simulink model "cell_station_2017_327_constant_load_for_battery_limit_suc"  (R2016b)
settings: Solver=VariableStepAuto  StartTime=0.0  StopTime=120*2  FixedStep=1e-6  RelTol=1e-3
undefined symbols (not defined in the file or in its folder): Acid, Lead, magnitude
libraries: powerlib x33, simulink x16, electricdrivelib x1
(part 1 of 2)
settings Model: Creator=Ray Hu  LastModifiedBy=Administrator

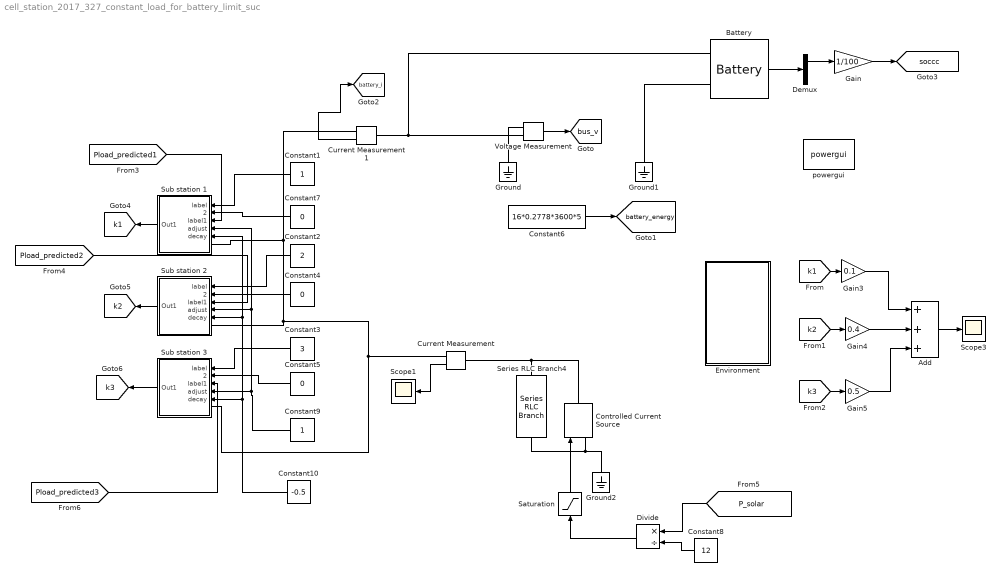
== system cell_station_2017_327_constant_load_for_battery_limit_suc ==
  Add : Sum  Inputs=+++
  Battery : electricdrivelib/Extra Sources/Battery  BatType=Lead-Acid  ShowTempParam=off  ThermalPreset=no  NomV=12  NomQ=0.2778*5  SOC=80  Batt_Tr=1  PresetModel=off  MaxQ=1.4469  MinV=9  FullV=13.0658  Dis_rate=10  R=0.086393  Normal_OP=0.2778*5  expZone="[12.2171      0.00463]"  current=[6.5 13 32.5]  Units=Time  Tci=20  NomT=25  T2=0  MaxQ2=2.208  FullV2=3.45  Normal_OP2=2.8  expZone2="[3.22        0.23]"  Rca=0.6  ti=1000  Dp=0
  Constant1 : Constant
  Constant10 : Constant  Value=-0.5
  Constant2 : Constant  Value=2
  Constant3 : Constant  Value=3
  Constant4 : Constant  Value=0
  Constant5 : Constant  Value=0
  Constant6 : Constant  Value=16*0.2778*3600*5
  Constant7 : Constant  Value=0
  Constant8 : Constant  Value=12
  Constant9 : Constant
  Controlled Current Source : powerlib/Electrical Sources/Controlled Current Source  Initialize=on  Source_Type=AC  Amplitude=0  Phase=0  Frequency=0  Measurements=None
  Current Measurement : powerlib/Measurements/Current Measurement  PhasorSimulation=off  OutputType=Complex  PSBequivalent=0
  Current Measurement1 : powerlib/Measurements/Current Measurement  PhasorSimulation=off  OutputType=Complex  PSBequivalent=0
  Demux : Demux  Outputs=3
  Divide : Product  Inputs=*/
  Environment : Subsystem
  Gain : Gain  Gain=1/100
  Gain3 : Gain  Gain=0.1
  Gain4 : Gain  Gain=0.4
  Gain5 : Gain  Gain=0.5
  Ground : powerlib/Elements/Ground  LConnTagsString=a
  Ground1 : powerlib/Elements/Ground  LConnTagsString=a
  Ground2 : powerlib/Elements/Ground  LConnTagsString=a
  Saturation : Saturate  UpperLimit=inf  LowerLimit=0
  Scope1 : Scope
  Scope3 : Scope
  Series RLC Branch4 : powerlib/Elements/Series RLC Branch  LConnTagsString=__new0  RConnTagsString=__new0  BranchType=C  Resistance=10  Inductance=1e-3  SetiL0=off  InitialCurrent=0  Capacitance=1e-6  Setx0=on  InitialVoltage=12  Measurements=None
  Sub station 1 : Subsystem
  Sub station 2 : Subsystem
  Sub station 3 : Subsystem
  Voltage Measurement : powerlib/Measurements/Voltage Measurement  PhasorSimulation=off  OutputType=Complex  PSBequivalent=0
  powergui : powerlib/powergui  Priority=1  SimulationMode=Continuous  SolverType=Tustin/Backward Euler (TBE)  SampleTime=50e-5  frequency=60  SPID=off  DisableSnubberDevices=off  DisableRonSwitches=off  DisableVfSwitches=off  SwTol=0  DisplayEquations=off  Interpol=off  ExternalGateDelay=off  methode=off  Ts=10  FunctionMessages=off  echomessages=off  HookPort=off  EnableUseOfTLC=off  x0status=blocks  frequencyindice=0  Pbase=100e6  ErrMax=1e-4  Iterations=50  UnitsV=kV  UnitsW=MW  buscounter=0  RestoreLinks=warning  ResistiveCurrentMeasurement=off  Frange=[0:2:500]  Ylog=off  Xlog=on  ShowGrid=off  save=off  variable=ZData  structure=0  ZoomFFT=off  StartTime=0.0  cycles=1  DisplayStyle=1  fundamental=60  FreqAxis=off  MaxFrequency=1000  frequencyindicesteady=1  RmsSteady=1  display=off
  tag scope: battery_energy=global, battery_i=global, bus_v=global, k1=global, k2=global, k3=global, soccc=global
  wires:
  Current Measurement/1 -> Scope1/1
  Voltage Measurement/1 -> [bus_v]
  Current Measurement1/1 -> [battery_i]
  Constant1/1 -> Sub station 1/1(label)
  Constant2/1 -> Sub station 2/1(label)
  Constant3/1 -> Sub station 3/1(label)
  Demux/1 -> Gain/1
  Constant4/1 -> Sub station 2/2(test_sig)
  Constant5/1 -> Sub station 3/2(test_sig)
  Constant6/1 -> [battery_energy]
  [k3] -> Gain5/1
  [k2] -> Gain4/1
  [k1] -> Gain3/1
  Gain4/1 -> Add/2
  Gain3/1 -> Add/1
  Gain5/1 -> Add/3
  Add/1 -> Scope3/1
  Constant7/1 -> Sub station 1/2(test_sig)
  Battery/1 -> Demux/1
  Sub station 1/1(Out1) -> [k1]
  Sub station 2/1(Out1) -> [k2]
  Sub station 3/1(Out1) -> [k3]
  [P_solar] -> Divide/1
  Constant8/1 -> Divide/2
  Divide/1 -> Saturation/1
  Saturation/1 -> Controlled Current Source/1
  [Pload_predicted1] -> Sub station 1/3(label1)
  [Pload_predicted2] -> Sub station 2/3(label1)
  [Pload_predicted3] -> Sub station 3/3(label1)
  Constant9/1 -> Sub station 3/4(adjust), Sub station 2/4(adjust), Sub station 1/4(adjust)
  Constant10/1 -> Sub station 3/5(decay), Sub station 2/5(decay), Sub station 1/5(decay)
  Gain/1 -> [soccc]
  connections:
  Voltage Measurement/LConn2 -- Ground/LConn1
  Current Measurement/RConn1 -- Sub station 3/LConn1 -- Sub station 2/LConn1 -- Sub station 1/LConn1 -- Current Measurement1/RConn1
  Controlled Current Source/RConn1 -- Series RLC Branch4/LConn1 -- Current Measurement/LConn1
  Ground1/LConn1 -- Battery/LConn2
  Current Measurement1/LConn1 -- Battery/LConn1 -- Voltage Measurement/LConn1
  Ground2/LConn1 -- Series RLC Branch4/RConn1 -- Controlled Current Source/LConn1

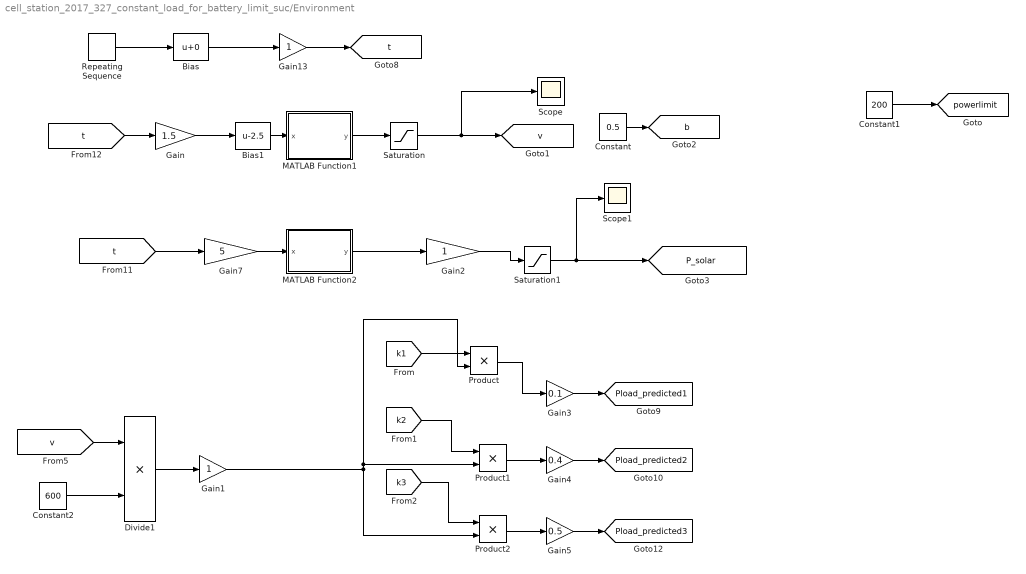
== system cell_station_2017_327_constant_load_for_battery_limit_suc/Environment ==
  Bias : Bias
  Bias1 : Bias  Bias=-2.5
  Constant : Constant  Value=0.5
  Constant1 : Constant  Value=200
  Constant2 : Constant  Value=600
  Divide1 : Product  Inputs=**
  Gain : Gain  Gain=1.5
  Gain1 : Gain
  Gain13 : Gain
  Gain2 : Gain
  Gain3 : Gain  Gain=0.1
  Gain4 : Gain  Gain=0.4
  Gain5 : Gain  Gain=0.5
  Gain7 : Gain  Gain=5
  MATLAB Function1 : MATLAB Function  TreatAsAtomicUnit=on
  MATLAB Function2 : MATLAB Function  TreatAsAtomicUnit=on
  Product : Product
  Product1 : Product
  Product2 : Product
  Repeating Sequence : simulink/Sources/Repeating Sequence  rep_seq_t=[0 120]  rep_seq_y=[0 24]
  Saturation : Saturate  UpperLimit=1  LowerLimit=0
  Saturation1 : Saturate  UpperLimit=inf  LowerLimit=0
  Scope : Scope
  Scope1 : Scope
  tag scope: P_solar=global, Pload_predicted1=global, Pload_predicted2=global, Pload_predicted3=global, b=global, powerlimit=global, t=global, v=global
  wires:
  Gain7/1 -> MATLAB Function2/1(x)
  MATLAB Function2/1(y) -> Gain2/1
  Bias/1 -> Gain13/1
  Saturation1/1 -> [P_solar], Scope1/1
  Gain13/1 -> [t]
  Repeating Sequence/1 -> Bias/1
  [t] -> Gain7/1
  MATLAB Function1/1(y) -> Saturation/1
  Gain/1 -> Bias1/1
  [t] -> Gain/1
  [v] -> Divide1/1
  Constant2/1 -> Divide1/2
  Divide1/1 -> Gain1/1
  Gain1/1 -> Product2/2, Product/2, Product1/2
  Gain3/1 -> [Pload_predicted1]
  Gain4/1 -> [Pload_predicted2]
  Gain5/1 -> [Pload_predicted3]
  Saturation/1 -> Scope/1, [v]
  Constant/1 -> [b]
  [k1] -> Product/1
  Product/1 -> Gain3/1
  [k3] -> Product2/1
  Product2/1 -> Gain5/1
  Product1/1 -> Gain4/1
  [k2] -> Product1/1
  Gain2/1 -> Saturation1/1
  Constant1/1 -> [powerlimit]
  Bias1/1 -> MATLAB Function1/1(x)

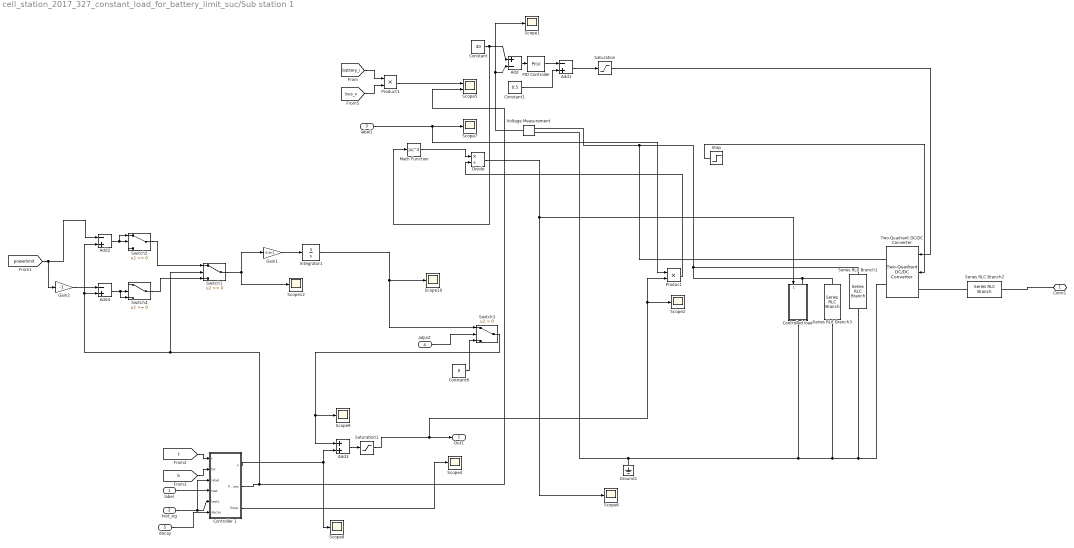
== system cell_station_2017_327_constant_load_for_battery_limit_suc/Sub station 1 ==
  label : Inport
  test_sig : Inport  Port=2
  label1 : Inport  Port=3
  adjust : Inport  Port=4
  decay : Inport  Port=5
  Add : Sum  Inputs=+-
  Add1 : Sum  Inputs=-+
  Add2 : Sum  Inputs=-+
  Add3 : Sum
  Add4 : Sum  Inputs=-+
  Constant : Constant  Value=40
  Constant1 : Constant  Value=0.5
  Constant6 : Constant  Value=0
  Controlled load : Subsystem
  Controller 1 : Subsystem
  Divide : Product  Inputs=*/
  Gain1 : Gain  Gain=-0.5e-2
  Gain2 : Gain  Gain=-1
  Ground1 : powerlib/Elements/Ground  LConnTagsString=a
  Integrator1 : Integrator
  Math Function : Math  Operator=magnitude^2  SaturateOnIntegerOverflow=on
  PID Controller : simulink/Continuous/PID Controller  Controller=PI  TimeDomain=Continuous-time  SampleTime=-1  IntegratorMethod=Forward Euler  FilterMethod=Forward Euler  Form=Parallel  UseFilter=on  ControllerParametersSource=internal  P=1e-5  I=0.1  D=0  N=100  InitialConditionSource=internal  InitialConditionForIntegrator=0  InitialConditionForFilter=0  ExternalReset=none  LimitOutput=off  UpperSaturationLimit=inf  LowerSaturationLimit=-inf  LinearizeAsGain=on  AntiWindupMode=none  Kb=1  TrackingMode=off  Kt=1  PParamMin=[]  PParamMax=[]  IParamMin=[]  IParamMax=[]  DParamMin=[]  DParamMax=[]  NParamMin=[]  NParamMax=[]  KbParamMin=[]  KbParamMax=[]  KtParamMin=[]  KtParamMax=[]  POutMin=[]  POutMax=[]  IOutMin=[]  IOutMax=[]  DOutMin=[]  DOutMax=[]  NOutMin=[]  NOutMax=[]  KbOutMin=[]  KbOutMax=[]  KtOutMin=[]  KtOutMax=[]  IntegratorOutMin=[]  IntegratorOutMax=[]  FilterOutMin=[]  FilterOutMax=[]  SumOutMin=[]  SumOutMax=[]  SumI1OutMin=[]  SumI1OutMax=[]  SumI2OutMin=[]  SumI2OutMax=[]  SumI3OutMin=[]  SumI3OutMax=[]  SumDOutMin=[]  SumDOutMax=[]  SaturationOutMin=[]  SaturationOutMax=[]  IntegratorContinuousStateAttributes=''  IntegratorStateMustResolveToSignalObject=off  IntegratorRTWStateStorageClass=Auto  FilterContinuousStateAttributes=''  FilterStateMustResolveToSignalObject=off  FilterRTWStateStorageClass=Auto  DifferentiatorICPrevScaledInput=0  DifferentiatorOutMin=[]  DifferentiatorOutMax=[]
  Product : Product
  Product1 : Product
  Saturation : Saturate  UpperLimit=0.9  LowerLimit=0.1
  Saturation1 : Saturate  UpperLimit=1  LowerLimit=0.1
  Scope{1..2,4,6..10,12} (9 alike) : Scope
  Scope5 : Scope  NumInputPorts=2
  Series RLC Branch1 : powerlib/Elements/Series RLC Branch  LConnTagsString=__new0  RConnTagsString=__new0  BranchType=C  Resistance=10  Inductance=1e-3  SetiL0=off  InitialCurrent=0  Capacitance=1e-6  Setx0=on  InitialVoltage=20  Measurements=None
  Series RLC Branch2 : powerlib/Elements/Series RLC Branch  LConnTagsString=__new0  RConnTagsString=__new0  BranchType=L  Resistance=10  Inductance=1e-3  SetiL0=off  InitialCurrent=0  Capacitance=1e-6  Setx0=off  InitialVoltage=0  Measurements=None
  Series RLC Branch3 : powerlib/Elements/Series RLC Branch  LConnTagsString=__new0  RConnTagsString=__new0  BranchType=R  Resistance=100  Inductance=1e-3  SetiL0=off  InitialCurrent=0  Capacitance=1e-6  Setx0=on  InitialVoltage=60  Measurements=None
  Step : Step  Time=0  Before=1  After=0  SampleTime=0
  Switch1 : Switch
  Switch2 : Switch
  Switch3 : Switch  Criteria=u2 > Threshold
  Switch4 : Switch
  Two-Quadrant DC/DC Converter : powerlib/Power Electronics/Two-Quadrant DC//DC Converter  ModelType=Average model (D-controlled)  Ron=1e-3  Rs=1e6  Cs=inf  Vforward=[0,0]  Ron_Diode=1e-3  Rs_Diode=1e6  Cs_Diode=inf  Vf_Diode=1e-3  Rs_CurrentSource=inf
  Voltage Measurement : powerlib/Measurements/Voltage Measurement  PhasorSimulation=off  OutputType=Complex  PSBequivalent=0
  Conn1 : PMIOPort  Port=1  Side=Left
  Out1 : Outport
  wires:
  Add1/1 -> Saturation/1
  Constant1/1 -> Add1/2
  PID Controller/1 -> Add1/1
  Step/1 -> Two-Quadrant DC/DC Converter/2
  Saturation/1 -> Two-Quadrant DC/DC Converter/1
  Add/1 -> PID Controller/1
  Voltage Measurement/1 -> Scope1/1, Add/2
  label1/1 -> Product/1, Scope7/1
  Product/1 -> Divide/2
  [t] -> Controller 1/1(t)
  [b] -> Controller 1/2(b0)
  label/1 -> Controller 1/3(label)
  Controller 1/3(Estar) -> Scope4/1
  Divide/1 -> Controlled load/1(Controllerd_R), Scope6/1
  Math Function/1 -> Divide/1
  Constant/1 -> Math Function/1, Add/1
  [battery_i] -> Product1/1
  [bus_v] -> Product1/2
  Product1/1 -> Scope5/1
  test_sig/1 -> Controller 1/5(test1), Controller 1/4(test)
  Controller 1/1("k ") -> Scope8/1, Add3/2
  Add3/1 -> Saturation1/1
  Saturation1/1 -> Product/2, Scope2/1, Out1/1
  decay/1 -> Controller 1/6(decay)
  Switch3/1 -> Scope9/1, Add3/1
  Gain1/1 -> Integrator1/1
  adjust/1 -> Switch3/2
  Integrator1/1 -> Switch3/1, Scope10/1
  [powerlimit] -> Gain2/1, Add2/1
  Switch1/1 -> Gain1/1, Scope12/1
  Constant6/1 -> Switch3/3
  Switch2/1 -> Switch1/1
  Switch4/1 -> Switch1/3
  Gain2/1 -> Add4/1
  Controller 1/2(P_guess) -> Switch1/2, Add2/2, Add4/2, Scope5/2
  Add2/1 -> Switch2/1, Switch2/2
  Add4/1 -> Switch4/3, Switch4/2
  connections:
  Conn1/RConn1 -- Series RLC Branch2/LConn1
  Series RLC Branch1/RConn1 -- Voltage Measurement/LConn2 -- Ground1/LConn1 -- Controlled load/RConn1 -- Series RLC Branch3/RConn1 -- Two-Quadrant DC/DC Converter/RConn2
  Series RLC Branch2/RConn1 -- Two-Quadrant DC/DC Converter/LConn1
  Series RLC Branch1/LConn1 -- Controlled load/LConn1 -- Series RLC Branch3/LConn1 -- Voltage Measurement/LConn1 -- Two-Quadrant DC/DC Converter/RConn1

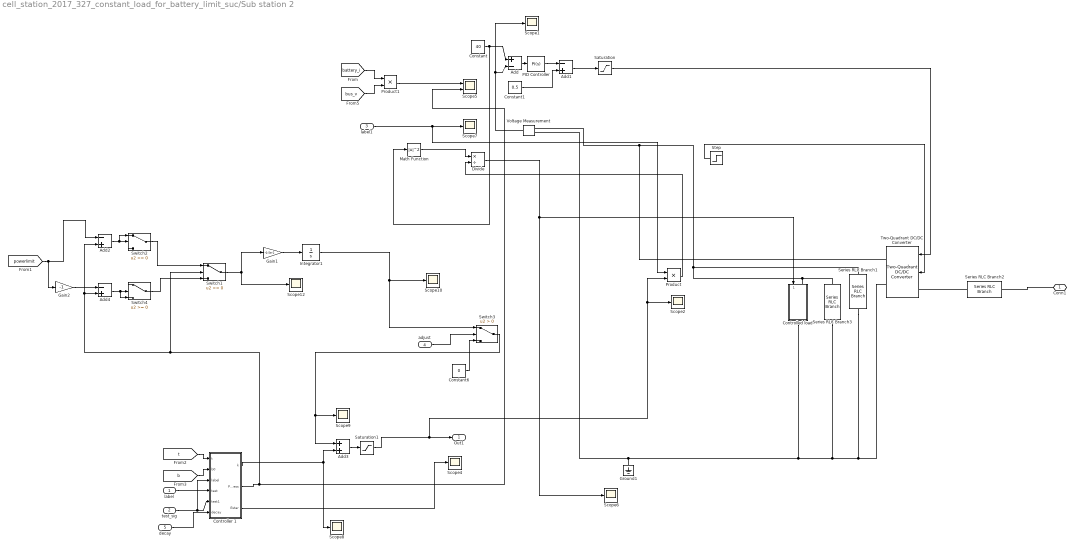
== system cell_station_2017_327_constant_load_for_battery_limit_suc/Sub station 2 ==
  label : Inport
  test_sig : Inport  Port=2
  label1 : Inport  Port=3
  adjust : Inport  Port=4
  decay : Inport  Port=5
  Add : Sum  Inputs=+-
  Add1 : Sum  Inputs=-+
  Add2 : Sum  Inputs=-+
  Add3 : Sum
  Add4 : Sum  Inputs=-+
  Constant : Constant  Value=40
  Constant1 : Constant  Value=0.5
  Constant6 : Constant  Value=0
  Controlled load : Subsystem
  Controller 1 : Subsystem
  Divide : Product  Inputs=*/
  Gain1 : Gain  Gain=-0.5e-2
  Gain2 : Gain  Gain=-1
  Ground1 : powerlib/Elements/Ground  LConnTagsString=a
  Integrator1 : Integrator
  Math Function : Math  Operator=magnitude^2  SaturateOnIntegerOverflow=on
  PID Controller : simulink/Continuous/PID Controller  Controller=PI  TimeDomain=Continuous-time  SampleTime=-1  IntegratorMethod=Forward Euler  FilterMethod=Forward Euler  Form=Parallel  UseFilter=on  ControllerParametersSource=internal  P=1e-5  I=0.1  D=0  N=100  InitialConditionSource=internal  InitialConditionForIntegrator=0  InitialConditionForFilter=0  ExternalReset=none  LimitOutput=off  UpperSaturationLimit=inf  LowerSaturationLimit=-inf  LinearizeAsGain=on  AntiWindupMode=none  Kb=1  TrackingMode=off  Kt=1  PParamMin=[]  PParamMax=[]  IParamMin=[]  IParamMax=[]  DParamMin=[]  DParamMax=[]  NParamMin=[]  NParamMax=[]  KbParamMin=[]  KbParamMax=[]  KtParamMin=[]  KtParamMax=[]  POutMin=[]  POutMax=[]  IOutMin=[]  IOutMax=[]  DOutMin=[]  DOutMax=[]  NOutMin=[]  NOutMax=[]  KbOutMin=[]  KbOutMax=[]  KtOutMin=[]  KtOutMax=[]  IntegratorOutMin=[]  IntegratorOutMax=[]  FilterOutMin=[]  FilterOutMax=[]  SumOutMin=[]  SumOutMax=[]  SumI1OutMin=[]  SumI1OutMax=[]  SumI2OutMin=[]  SumI2OutMax=[]  SumI3OutMin=[]  SumI3OutMax=[]  SumDOutMin=[]  SumDOutMax=[]  SaturationOutMin=[]  SaturationOutMax=[]  IntegratorContinuousStateAttributes=''  IntegratorStateMustResolveToSignalObject=off  IntegratorRTWStateStorageClass=Auto  FilterContinuousStateAttributes=''  FilterStateMustResolveToSignalObject=off  FilterRTWStateStorageClass=Auto  DifferentiatorICPrevScaledInput=0  DifferentiatorOutMin=[]  DifferentiatorOutMax=[]
  Product : Product
  Product1 : Product
  Saturation : Saturate  UpperLimit=0.9  LowerLimit=0.1
  Saturation1 : Saturate  UpperLimit=1  LowerLimit=0.1
  Scope{1..2,4,6..10,12} (9 alike) : Scope
  Scope5 : Scope  NumInputPorts=2
  Series RLC Branch1 : powerlib/Elements/Series RLC Branch  LConnTagsString=__new0  RConnTagsString=__new0  BranchType=C  Resistance=10  Inductance=1e-3  SetiL0=off  InitialCurrent=0  Capacitance=1e-6  Setx0=on  InitialVoltage=20  Measurements=None
  Series RLC Branch2 : powerlib/Elements/Series RLC Branch  LConnTagsString=__new0  RConnTagsString=__new0  BranchType=L  Resistance=10  Inductance=1e-3  SetiL0=off  InitialCurrent=0  Capacitance=1e-6  Setx0=off  InitialVoltage=0  Measurements=None
  Series RLC Branch3 : powerlib/Elements/Series RLC Branch  LConnTagsString=__new0  RConnTagsString=__new0  BranchType=R  Resistance=100  Inductance=1e-3  SetiL0=off  InitialCurrent=0  Capacitance=1e-6  Setx0=on  InitialVoltage=60  Measurements=None
  Step : Step  Time=0  Before=1  After=0  SampleTime=0
  Switch1 : Switch
  Switch2 : Switch
  Switch3 : Switch  Criteria=u2 > Threshold
  Switch4 : Switch
  Two-Quadrant DC/DC Converter : powerlib/Power Electronics/Two-Quadrant DC//DC Converter  ModelType=Average model (D-controlled)  Ron=1e-3  Rs=1e6  Cs=inf  Vforward=[0,0]  Ron_Diode=1e-3  Rs_Diode=1e6  Cs_Diode=inf  Vf_Diode=1e-3  Rs_CurrentSource=inf
  Voltage Measurement : powerlib/Measurements/Voltage Measurement  PhasorSimulation=off  OutputType=Complex  PSBequivalent=0
  Conn1 : PMIOPort  Port=1  Side=Left
  Out1 : Outport
  wires:
  Add1/1 -> Saturation/1
  Constant1/1 -> Add1/2
  PID Controller/1 -> Add1/1
  Step/1 -> Two-Quadrant DC/DC Converter/2
  Saturation/1 -> Two-Quadrant DC/DC Converter/1
  Add/1 -> PID Controller/1
  Voltage Measurement/1 -> Scope1/1, Add/2
  label1/1 -> Product/1, Scope7/1
  Product/1 -> Divide/2
  [t] -> Controller 1/1(t)
  [b] -> Controller 1/2(b0)
  label/1 -> Controller 1/3(label)
  Controller 1/3(Estar) -> Scope4/1
  Divide/1 -> Controlled load/1(Controllerd_R), Scope6/1
  Math Function/1 -> Divide/1
  Constant/1 -> Math Function/1, Add/1
  [battery_i] -> Product1/1
  [bus_v] -> Product1/2
  Product1/1 -> Scope5/1
  test_sig/1 -> Controller 1/5(test1), Controller 1/4(test)
  Controller 1/1("k ") -> Scope8/1, Add3/2
  Add3/1 -> Saturation1/1
  Saturation1/1 -> Product/2, Scope2/1, Out1/1
  decay/1 -> Controller 1/6(decay)
  Switch3/1 -> Scope9/1, Add3/1
  Gain1/1 -> Integrator1/1
  adjust/1 -> Switch3/2
  Integrator1/1 -> Switch3/1, Scope10/1
  [powerlimit] -> Gain2/1, Add2/1
  Switch1/1 -> Gain1/1, Scope12/1
  Constant6/1 -> Switch3/3
  Switch2/1 -> Switch1/1
  Switch4/1 -> Switch1/3
  Gain2/1 -> Add4/1
  Controller 1/2(P_guess) -> Switch1/2, Add2/2, Add4/2, Scope5/2
  Add2/1 -> Switch2/1, Switch2/2
  Add4/1 -> Switch4/3, Switch4/2
  connections:
  Conn1/RConn1 -- Series RLC Branch2/LConn1
  Series RLC Branch1/RConn1 -- Voltage Measurement/LConn2 -- Ground1/LConn1 -- Controlled load/RConn1 -- Series RLC Branch3/RConn1 -- Two-Quadrant DC/DC Converter/RConn2
  Series RLC Branch2/RConn1 -- Two-Quadrant DC/DC Converter/LConn1
  Series RLC Branch1/LConn1 -- Controlled load/LConn1 -- Series RLC Branch3/LConn1 -- Voltage Measurement/LConn1 -- Two-Quadrant DC/DC Converter/RConn1

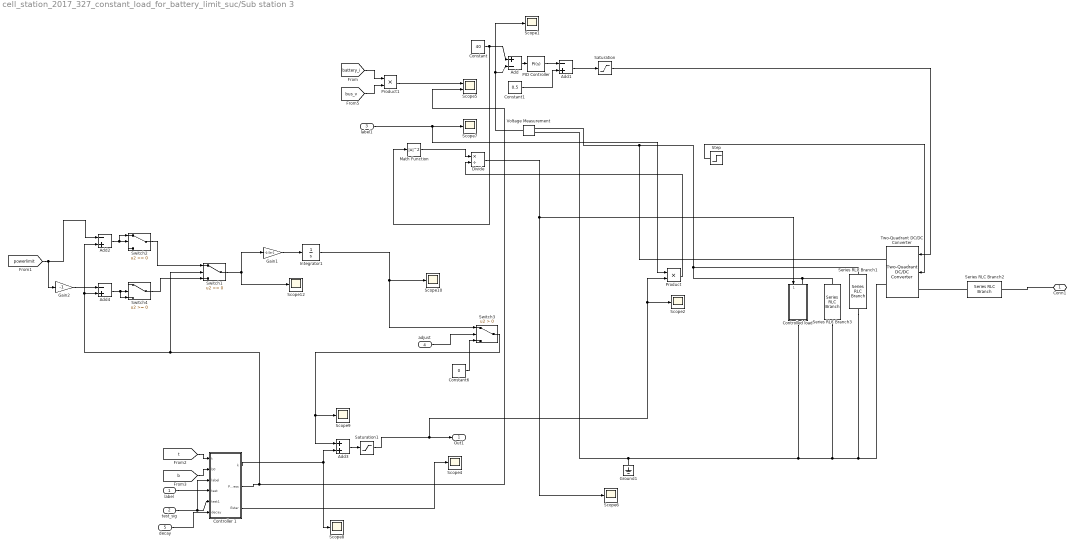
== system cell_station_2017_327_constant_load_for_battery_limit_suc/Sub station 3 ==
  label : Inport
  test_sig : Inport  Port=2
  label1 : Inport  Port=3
  adjust : Inport  Port=4
  decay : Inport  Port=5
  Add : Sum  Inputs=+-
  Add1 : Sum  Inputs=-+
  Add2 : Sum  Inputs=-+
  Add3 : Sum
  Add4 : Sum  Inputs=-+
  Constant : Constant  Value=40
  Constant1 : Constant  Value=0.5
  Constant6 : Constant  Value=0
  Controlled load : Subsystem
  Controller 1 : Subsystem
  Divide : Product  Inputs=*/
  Gain1 : Gain  Gain=-0.5e-2
  Gain2 : Gain  Gain=-1
  Ground1 : powerlib/Elements/Ground  LConnTagsString=a
  Integrator1 : Integrator
  Math Function : Math  Operator=magnitude^2  SaturateOnIntegerOverflow=on
  PID Controller : simulink/Continuous/PID Controller  Controller=PI  TimeDomain=Continuous-time  SampleTime=-1  IntegratorMethod=Forward Euler  FilterMethod=Forward Euler  Form=Parallel  UseFilter=on  ControllerParametersSource=internal  P=1e-5  I=0.1  D=0  N=100  InitialConditionSource=internal  InitialConditionForIntegrator=0  InitialConditionForFilter=0  ExternalReset=none  LimitOutput=off  UpperSaturationLimit=inf  LowerSaturationLimit=-inf  LinearizeAsGain=on  AntiWindupMode=none  Kb=1  TrackingMode=off  Kt=1  PParamMin=[]  PParamMax=[]  IParamMin=[]  IParamMax=[]  DParamMin=[]  DParamMax=[]  NParamMin=[]  NParamMax=[]  KbParamMin=[]  KbParamMax=[]  KtParamMin=[]  KtParamMax=[]  POutMin=[]  POutMax=[]  IOutMin=[]  IOutMax=[]  DOutMin=[]  DOutMax=[]  NOutMin=[]  NOutMax=[]  KbOutMin=[]  KbOutMax=[]  KtOutMin=[]  KtOutMax=[]  IntegratorOutMin=[]  IntegratorOutMax=[]  FilterOutMin=[]  FilterOutMax=[]  SumOutMin=[]  SumOutMax=[]  SumI1OutMin=[]  SumI1OutMax=[]  SumI2OutMin=[]  SumI2OutMax=[]  SumI3OutMin=[]  SumI3OutMax=[]  SumDOutMin=[]  SumDOutMax=[]  SaturationOutMin=[]  SaturationOutMax=[]  IntegratorContinuousStateAttributes=''  IntegratorStateMustResolveToSignalObject=off  IntegratorRTWStateStorageClass=Auto  FilterContinuousStateAttributes=''  FilterStateMustResolveToSignalObject=off  FilterRTWStateStorageClass=Auto  DifferentiatorICPrevScaledInput=0  DifferentiatorOutMin=[]  DifferentiatorOutMax=[]
  Product : Product
  Product1 : Product
  Saturation : Saturate  UpperLimit=0.9  LowerLimit=0.1
  Saturation1 : Saturate  UpperLimit=1  LowerLimit=0.1
  Scope{1..2,4,6..10,12} (9 alike) : Scope
  Scope5 : Scope  NumInputPorts=2
  Series RLC Branch1 : powerlib/Elements/Series RLC Branch  LConnTagsString=__new0  RConnTagsString=__new0  BranchType=C  Resistance=10  Inductance=1e-3  SetiL0=off  InitialCurrent=0  Capacitance=1e-6  Setx0=on  InitialVoltage=20  Measurements=None
  Series RLC Branch2 : powerlib/Elements/Series RLC Branch  LConnTagsString=__new0  RConnTagsString=__new0  BranchType=L  Resistance=10  Inductance=1e-3  SetiL0=off  InitialCurrent=0  Capacitance=1e-6  Setx0=off  InitialVoltage=0  Measurements=None
  Series RLC Branch3 : powerlib/Elements/Series RLC Branch  LConnTagsString=__new0  RConnTagsString=__new0  BranchType=R  Resistance=100  Inductance=1e-3  SetiL0=off  InitialCurrent=0  Capacitance=1e-6  Setx0=on  InitialVoltage=60  Measurements=None
  Step : Step  Time=0  Before=1  After=0  SampleTime=0
  Switch1 : Switch
  Switch2 : Switch
  Switch3 : Switch  Criteria=u2 > Threshold
  Switch4 : Switch
  Two-Quadrant DC/DC Converter : powerlib/Power Electronics/Two-Quadrant DC//DC Converter  ModelType=Average model (D-controlled)  Ron=1e-3  Rs=1e6  Cs=inf  Vforward=[0,0]  Ron_Diode=1e-3  Rs_Diode=1e6  Cs_Diode=inf  Vf_Diode=1e-3  Rs_CurrentSource=inf
  Voltage Measurement : powerlib/Measurements/Voltage Measurement  PhasorSimulation=off  OutputType=Complex  PSBequivalent=0
  Conn1 : PMIOPort  Port=1  Side=Left
  Out1 : Outport
  wires:
  Add1/1 -> Saturation/1
  Constant1/1 -> Add1/2
  PID Controller/1 -> Add1/1
  Step/1 -> Two-Quadrant DC/DC Converter/2
  Saturation/1 -> Two-Quadrant DC/DC Converter/1
  Add/1 -> PID Controller/1
  Voltage Measurement/1 -> Scope1/1, Add/2
  label1/1 -> Product/1, Scope7/1
  Product/1 -> Divide/2
  [t] -> Controller 1/1(t)
  [b] -> Controller 1/2(b0)
  label/1 -> Controller 1/3(label)
  Controller 1/3(Estar) -> Scope4/1
  Divide/1 -> Controlled load/1(Controllerd_R), Scope6/1
  Math Function/1 -> Divide/1
  Constant/1 -> Math Function/1, Add/1
  [battery_i] -> Product1/1
  [bus_v] -> Product1/2
  Product1/1 -> Scope5/1
  test_sig/1 -> Controller 1/5(test1), Controller 1/4(test)
  Controller 1/1("k ") -> Scope8/1, Add3/2
  Add3/1 -> Saturation1/1
  Saturation1/1 -> Product/2, Scope2/1, Out1/1
  decay/1 -> Controller 1/6(decay)
  Switch3/1 -> Scope9/1, Add3/1
  Gain1/1 -> Integrator1/1
  adjust/1 -> Switch3/2
  Integrator1/1 -> Switch3/1, Scope10/1
  [powerlimit] -> Gain2/1, Add2/1
  Switch1/1 -> Gain1/1, Scope12/1
  Constant6/1 -> Switch3/3
  Switch2/1 -> Switch1/1
  Switch4/1 -> Switch1/3
  Gain2/1 -> Add4/1
  Controller 1/2(P_guess) -> Switch1/2, Add2/2, Add4/2, Scope5/2
  Add2/1 -> Switch2/1, Switch2/2
  Add4/1 -> Switch4/3, Switch4/2
  connections:
  Conn1/RConn1 -- Series RLC Branch2/LConn1
  Series RLC Branch1/RConn1 -- Voltage Measurement/LConn2 -- Ground1/LConn1 -- Controlled load/RConn1 -- Series RLC Branch3/RConn1 -- Two-Quadrant DC/DC Converter/RConn2
  Series RLC Branch2/RConn1 -- Two-Quadrant DC/DC Converter/LConn1
  Series RLC Branch1/LConn1 -- Controlled load/LConn1 -- Series RLC Branch3/LConn1 -- Voltage Measurement/LConn1 -- Two-Quadrant DC/DC Converter/RConn1

== system cell_station_2017_327_constant_load_for_battery_limit_suc/Sub station 1/Controlled load ==
  Controllerd_R : Inport
  Controlled Current Source : powerlib/Electrical Sources/Controlled Current Source  Initialize=on  Source_Type=DC  Amplitude=0  Phase=0  Frequency=0  Measurements=None
  Divide : Product  Inputs=*/
  Saturation : Saturate  UpperLimit=inf  LowerLimit=0.1
  Voltage Measurement : powerlib/Measurements/Voltage Measurement  PhasorSimulation=off  OutputType=Complex  PSBequivalent=0
  Conn1 : PMIOPort  Port=1  Side=Left
  Conn2 : PMIOPort  Port=2  Side=Right
  wires:
  Voltage Measurement/1 -> Divide/1
  Controllerd_R/1 -> Saturation/1
  Divide/1 -> Controlled Current Source/1
  Saturation/1 -> Divide/2
  connections:
  Voltage Measurement/LConn2 -- Controlled Current Source/RConn1 -- Conn2/RConn1
  Voltage Measurement/LConn1 -- Controlled Current Source/LConn1 -- Conn1/RConn1

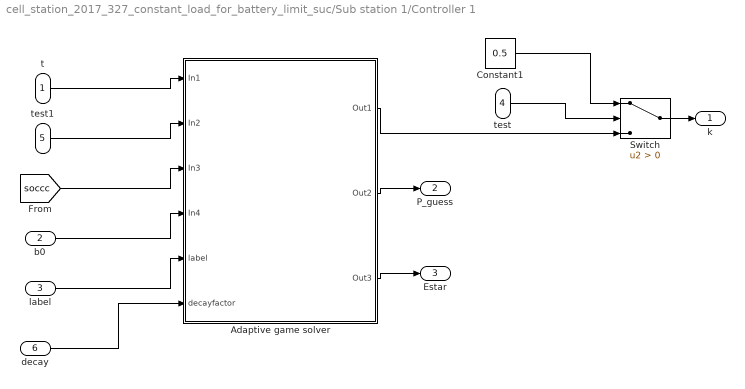
== system cell_station_2017_327_constant_load_for_battery_limit_suc/Sub station 1/Controller 1 ==
  t : Inport
  b0 : Inport  Port=2
  label : Inport  Port=3
  test : Inport  Port=4
  test1 : Inport  Port=5
  decay : Inport  Port=6
  Adaptive game solver : Subsystem
  Constant1 : Constant  Value=0.5
  Switch : Switch  Criteria=u2 > Threshold
  "k " : Outport
  P_guess : Outport  Port=2
  Estar : Outport  Port=3
  wires:
  Constant1/1 -> Switch/1
  Switch/1 -> "k "/1
  test/1 -> Switch/2
  t/1 -> Adaptive game solver/1(In1)
  test1/1 -> Adaptive game solver/2(In2)
  [soccc] -> Adaptive game solver/3(In3)
  b0/1 -> Adaptive game solver/4(In4)
  label/1 -> Adaptive game solver/5(label)
  Adaptive game solver/1(Out1) -> Switch/3
  Adaptive game solver/2(Out2) -> P_guess/1
  Adaptive game solver/3(Out3) -> Estar/1
  decay/1 -> Adaptive game solver/6(decayfactor)

== system cell_station_2017_327_constant_load_for_battery_limit_suc/Sub station 2/Controlled load ==
  Controllerd_R : Inport
  Controlled Current Source : powerlib/Electrical Sources/Controlled Current Source  Initialize=on  Source_Type=DC  Amplitude=0  Phase=0  Frequency=0  Measurements=None
  Divide : Product  Inputs=*/
  Saturation : Saturate  UpperLimit=inf  LowerLimit=0.1
  Voltage Measurement : powerlib/Measurements/Voltage Measurement  PhasorSimulation=off  OutputType=Complex  PSBequivalent=0
  Conn1 : PMIOPort  Port=1  Side=Left
  Conn2 : PMIOPort  Port=2  Side=Right
  wires:
  Voltage Measurement/1 -> Divide/1
  Controllerd_R/1 -> Saturation/1
  Divide/1 -> Controlled Current Source/1
  Saturation/1 -> Divide/2
  connections:
  Voltage Measurement/LConn2 -- Controlled Current Source/RConn1 -- Conn2/RConn1
  Voltage Measurement/LConn1 -- Controlled Current Source/LConn1 -- Conn1/RConn1

== system cell_station_2017_327_constant_load_for_battery_limit_suc/Sub station 2/Controller 1 ==
  t : Inport
  b0 : Inport  Port=2
  label : Inport  Port=3
  test : Inport  Port=4
  test1 : Inport  Port=5
  decay : Inport  Port=6
  Adaptive game solver : Subsystem
  Constant1 : Constant  Value=0.5
  Switch : Switch  Criteria=u2 > Threshold
  "k " : Outport
  P_guess : Outport  Port=2
  Estar : Outport  Port=3
  wires:
  Constant1/1 -> Switch/1
  Switch/1 -> "k "/1
  test/1 -> Switch/2
  t/1 -> Adaptive game solver/1(In1)
  test1/1 -> Adaptive game solver/2(In2)
  [soccc] -> Adaptive game solver/3(In3)
  b0/1 -> Adaptive game solver/4(In4)
  label/1 -> Adaptive game solver/5(label)
  Adaptive game solver/1(Out1) -> Switch/3
  Adaptive game solver/2(Out2) -> P_guess/1
  Adaptive game solver/3(Out3) -> Estar/1
  decay/1 -> Adaptive game solver/6(decayfactor)

== system cell_station_2017_327_constant_load_for_battery_limit_suc/Sub station 3/Controlled load ==
  Controllerd_R : Inport
  Controlled Current Source : powerlib/Electrical Sources/Controlled Current Source  Initialize=on  Source_Type=DC  Amplitude=0  Phase=0  Frequency=0  Measurements=None
  Divide : Product  Inputs=*/
  Saturation : Saturate  UpperLimit=inf  LowerLimit=0.1
  Voltage Measurement : powerlib/Measurements/Voltage Measurement  PhasorSimulation=off  OutputType=Complex  PSBequivalent=0
  Conn1 : PMIOPort  Port=1  Side=Left
  Conn2 : PMIOPort  Port=2  Side=Right
  wires:
  Voltage Measurement/1 -> Divide/1
  Controllerd_R/1 -> Saturation/1
  Divide/1 -> Controlled Current Source/1
  Saturation/1 -> Divide/2
  connections:
  Voltage Measurement/LConn2 -- Controlled Current Source/RConn1 -- Conn2/RConn1
  Voltage Measurement/LConn1 -- Controlled Current Source/LConn1 -- Conn1/RConn1

== system cell_station_2017_327_constant_load_for_battery_limit_suc/Sub station 3/Controller 1 ==
  t : Inport
  b0 : Inport  Port=2
  label : Inport  Port=3
  test : Inport  Port=4
  test1 : Inport  Port=5
  decay : Inport  Port=6
  Adaptive game solver : Subsystem
  Constant1 : Constant  Value=0.5
  Switch : Switch  Criteria=u2 > Threshold
  "k " : Outport
  P_guess : Outport  Port=2
  Estar : Outport  Port=3
  wires:
  Constant1/1 -> Switch/1
  Switch/1 -> "k "/1
  test/1 -> Switch/2
  t/1 -> Adaptive game solver/1(In1)
  test1/1 -> Adaptive game solver/2(In2)
  [soccc] -> Adaptive game solver/3(In3)
  b0/1 -> Adaptive game solver/4(In4)
  label/1 -> Adaptive game solver/5(label)
  Adaptive game solver/1(Out1) -> Switch/3
  Adaptive game solver/2(Out2) -> P_guess/1
  Adaptive game solver/3(Out3) -> Estar/1
  decay/1 -> Adaptive game solver/6(decayfactor)

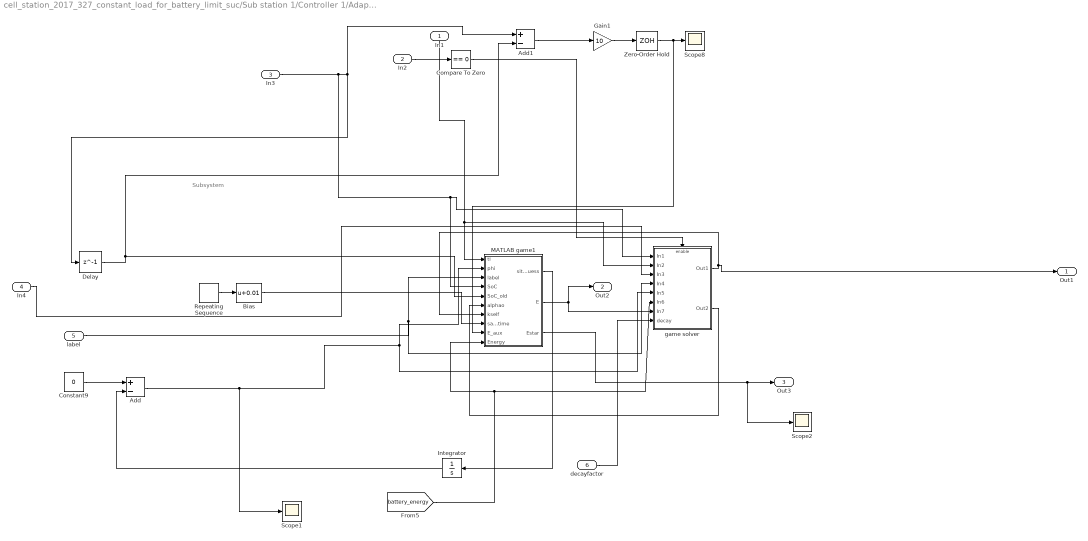
== system cell_station_2017_327_constant_load_for_battery_limit_suc/Sub station 1/Controller 1/Adaptive game solver ==
  note: Subsystem
  In1 : Inport
  In2 : Inport  Port=2
  In3 : Inport  Port=3
  In4 : Inport  Port=4
  label : Inport  Port=5
  decayfactor : Inport  Port=6
  Add : Sum  Inputs=+-
  Add1 : Sum  Inputs=+-
  Bias : Bias  Bias=0.01
  Compare To Zero : simulink/Logic and Bit Operations/Compare To Zero  relop===  OutDataTypeStr=boolean
  Constant9 : Constant  Value=0
  Delay : Delay  DelayLength=1  InitialCondition=0  SampleTime=0.1
  Gain1 : Gain  Gain=10
  Integrator : Integrator
  MATLAB game1 : MATLAB Function  TreatAsAtomicUnit=on
      settings: MinAlgLoopOccurrences=on
  Repeating Sequence : simulink/Sources/Repeating Sequence  rep_seq_t=[0 0.5]  rep_seq_y=[0 0.5]
  Scope1 : Scope
  Scope2 : Scope
  Scope8 : Scope
  Zero-Order Hold : ZeroOrderHold  SampleTime=0.1
  game solver : Subsystem
  Out1 : Outport
  Out2 : Outport  Port=2
  Out3 : Outport  Port=3
  wires:
  game solver/2(Out2) -> MATLAB game1/6(alphao)
  Constant9/1 -> Add/1
  Repeating Sequence/1 -> Bias/1
  Add1/1 -> Gain1/1
  Gain1/1 -> Zero-Order Hold/1
  In2/1 -> Compare To Zero/1
  Compare To Zero/1 -> game solver/Enable
  [battery_energy] -> MATLAB game1/10(Energy), game solver/6(In6)
  Bias/1 -> MATLAB game1/8(sampletime)
  label/1 -> game solver/4(In4), MATLAB game1/3(label)
  Add/1 -> Scope1/1, game solver/5(In5), MATLAB game1/2(phi)
  In1/1 -> MATLAB game1/1(ti), game solver/2(In2)
  In4/1 -> game solver/3(In3)
  Integrator/1 -> Add/2
  MATLAB game1/1(sitaguess) -> Integrator/1
  Delay/1 -> MATLAB game1/5(SoC_old), Add1/2
  Zero-Order Hold/1 -> MATLAB game1/9(E_aux), Scope8/1
  MATLAB game1/2(E) -> game solver/7(In7), Out2/1
  game solver/1(Out1) -> Out1/1, MATLAB game1/7(kself)
  In3/1 -> game solver/1(In1), MATLAB game1/4(SoC), Add1/1, Delay/1
  MATLAB game1/3(Estar) -> Scope2/1, Out3/1
  decayfactor/1 -> game solver/8(decay)

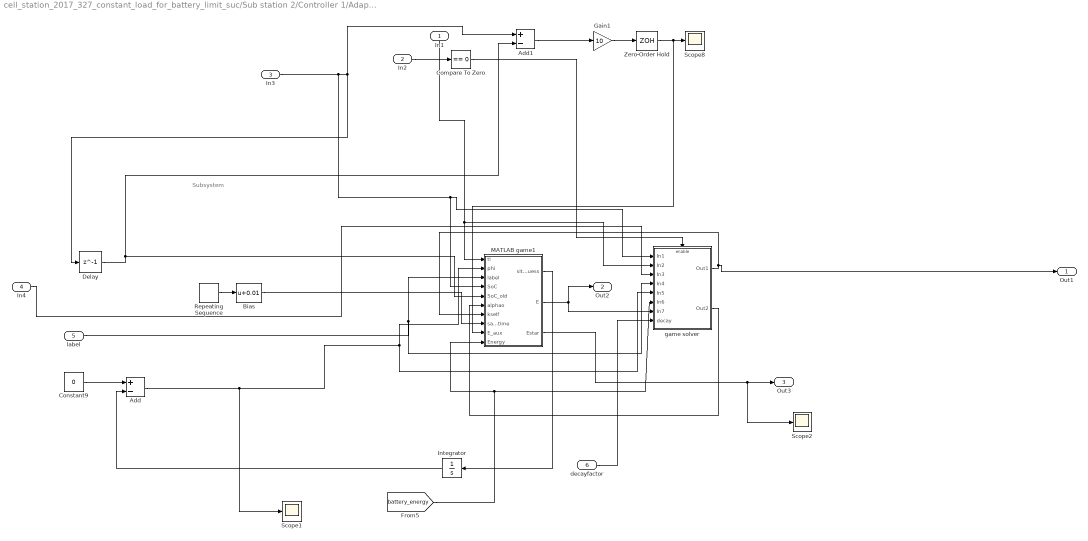
== system cell_station_2017_327_constant_load_for_battery_limit_suc/Sub station 2/Controller 1/Adaptive game solver ==
  note: Subsystem
  In1 : Inport
  In2 : Inport  Port=2
  In3 : Inport  Port=3
  In4 : Inport  Port=4
  label : Inport  Port=5
  decayfactor : Inport  Port=6
  Add : Sum  Inputs=+-
  Add1 : Sum  Inputs=+-
  Bias : Bias  Bias=0.01
  Compare To Zero : simulink/Logic and Bit Operations/Compare To Zero  relop===  OutDataTypeStr=boolean
  Constant9 : Constant  Value=0
  Delay : Delay  DelayLength=1  InitialCondition=0  SampleTime=0.1
  Gain1 : Gain  Gain=10
  Integrator : Integrator
  MATLAB game1 : MATLAB Function  TreatAsAtomicUnit=on
      settings: MinAlgLoopOccurrences=on
  Repeating Sequence : simulink/Sources/Repeating Sequence  rep_seq_t=[0 0.5]  rep_seq_y=[0 0.5]
  Scope1 : Scope
  Scope2 : Scope
  Scope8 : Scope
  Zero-Order Hold : ZeroOrderHold  SampleTime=0.1
  game solver : Subsystem
  Out1 : Outport
  Out2 : Outport  Port=2
  Out3 : Outport  Port=3
  wires:
  game solver/2(Out2) -> MATLAB game1/6(alphao)
  Constant9/1 -> Add/1
  Repeating Sequence/1 -> Bias/1
  Add1/1 -> Gain1/1
  Gain1/1 -> Zero-Order Hold/1
  In2/1 -> Compare To Zero/1
  Compare To Zero/1 -> game solver/Enable
  [battery_energy] -> MATLAB game1/10(Energy), game solver/6(In6)
  Bias/1 -> MATLAB game1/8(sampletime)
  label/1 -> game solver/4(In4), MATLAB game1/3(label)
  Add/1 -> Scope1/1, game solver/5(In5), MATLAB game1/2(phi)
  In1/1 -> MATLAB game1/1(ti), game solver/2(In2)
  In4/1 -> game solver/3(In3)
  Integrator/1 -> Add/2
  MATLAB game1/1(sitaguess) -> Integrator/1
  Delay/1 -> MATLAB game1/5(SoC_old), Add1/2
  Zero-Order Hold/1 -> MATLAB game1/9(E_aux), Scope8/1
  MATLAB game1/2(E) -> game solver/7(In7), Out2/1
  game solver/1(Out1) -> Out1/1, MATLAB game1/7(kself)
  In3/1 -> game solver/1(In1), MATLAB game1/4(SoC), Add1/1, Delay/1
  MATLAB game1/3(Estar) -> Scope2/1, Out3/1
  decayfactor/1 -> game solver/8(decay)

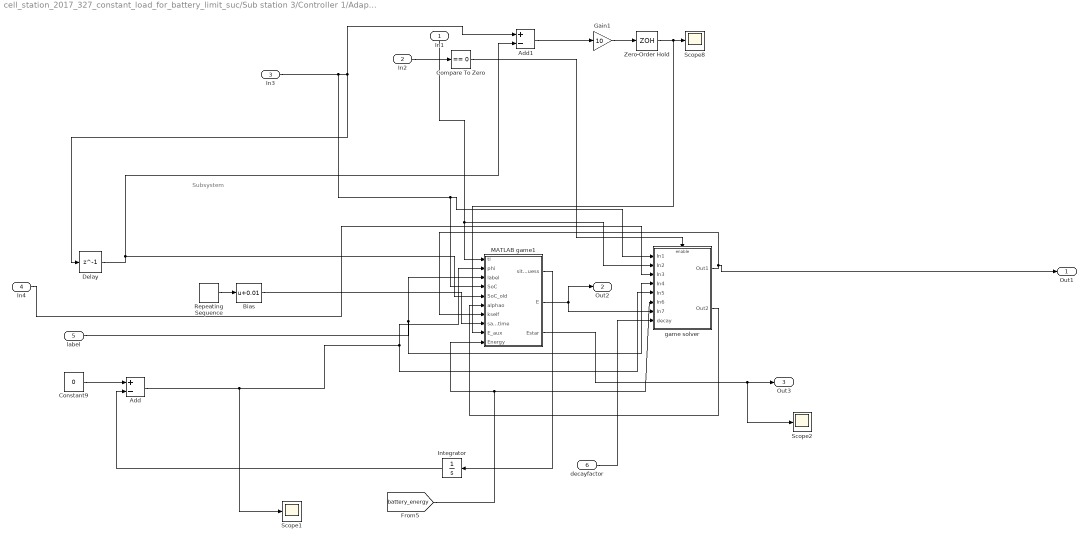
== system cell_station_2017_327_constant_load_for_battery_limit_suc/Sub station 3/Controller 1/Adaptive game solver ==
  note: Subsystem
  In1 : Inport
  In2 : Inport  Port=2
  In3 : Inport  Port=3
  In4 : Inport  Port=4
  label : Inport  Port=5
  decayfactor : Inport  Port=6
  Add : Sum  Inputs=+-
  Add1 : Sum  Inputs=+-
  Bias : Bias  Bias=0.01
  Compare To Zero : simulink/Logic and Bit Operations/Compare To Zero  relop===  OutDataTypeStr=boolean
  Constant9 : Constant  Value=0
  Delay : Delay  DelayLength=1  InitialCondition=0  SampleTime=0.1
  Gain1 : Gain  Gain=10
  Integrator : Integrator
  MATLAB game1 : MATLAB Function  TreatAsAtomicUnit=on
      settings: MinAlgLoopOccurrences=on
  Repeating Sequence : simulink/Sources/Repeating Sequence  rep_seq_t=[0 0.5]  rep_seq_y=[0 0.5]
  Scope1 : Scope
  Scope2 : Scope
  Scope8 : Scope
  Zero-Order Hold : ZeroOrderHold  SampleTime=0.1
  game solver : Subsystem
  Out1 : Outport
  Out2 : Outport  Port=2
  Out3 : Outport  Port=3
  wires:
  game solver/2(Out2) -> MATLAB game1/6(alphao)
  Constant9/1 -> Add/1
  Repeating Sequence/1 -> Bias/1
  Add1/1 -> Gain1/1
  Gain1/1 -> Zero-Order Hold/1
  In2/1 -> Compare To Zero/1
  Compare To Zero/1 -> game solver/Enable
  [battery_energy] -> MATLAB game1/10(Energy), game solver/6(In6)
  Bias/1 -> MATLAB game1/8(sampletime)
  label/1 -> game solver/4(In4), MATLAB game1/3(label)
  Add/1 -> Scope1/1, game solver/5(In5), MATLAB game1/2(phi)
  In1/1 -> MATLAB game1/1(ti), game solver/2(In2)
  In4/1 -> game solver/3(In3)
  Integrator/1 -> Add/2
  MATLAB game1/1(sitaguess) -> Integrator/1
  Delay/1 -> MATLAB game1/5(SoC_old), Add1/2
  Zero-Order Hold/1 -> MATLAB game1/9(E_aux), Scope8/1
  MATLAB game1/2(E) -> game solver/7(In7), Out2/1
  game solver/1(Out1) -> Out1/1, MATLAB game1/7(kself)
  In3/1 -> game solver/1(In1), MATLAB game1/4(SoC), Add1/1, Delay/1
  MATLAB game1/3(Estar) -> Scope2/1, Out3/1
  decayfactor/1 -> game solver/8(decay)

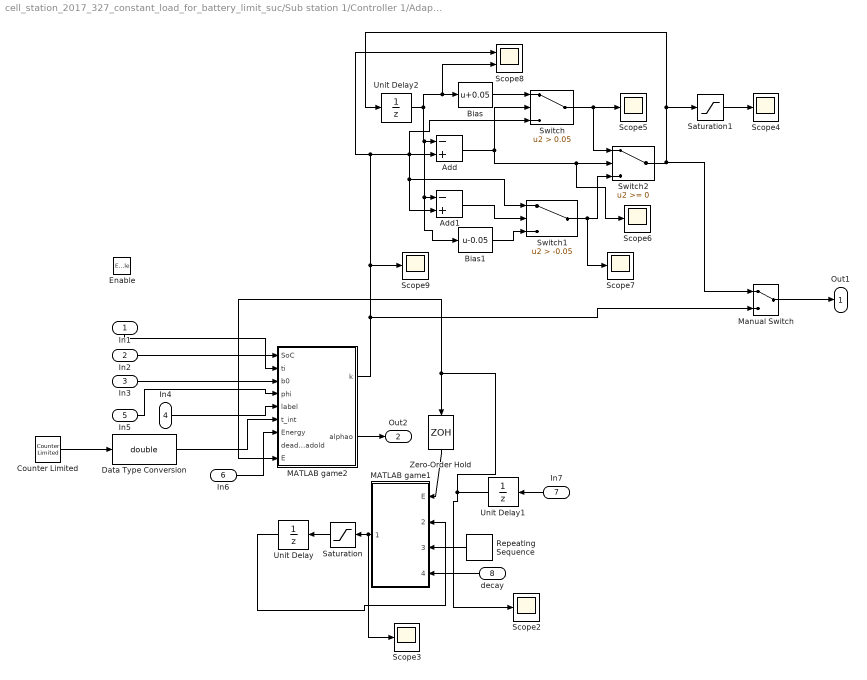
== system cell_station_2017_327_constant_load_for_battery_limit_suc/Sub station 1/Controller 1/Adaptive game solver/game solver ==
  In1 : Inport
  In2 : Inport  Port=2
  In3 : Inport  Port=3
  In4 : Inport  Port=4
  In5 : Inport  Port=5
  In6 : Inport  Port=6
  In7 : Inport  Port=7
  decay : Inport  Port=8
  Enable : EnablePort
  Add : Sum  Inputs=-+
  Add1 : Sum  Inputs=-+
  Bias : Bias  Bias=0.05
  Bias1 : Bias  Bias=-0.05
  Counter Limited : simulink/Sources/Counter Limited  uplimit=24  tsamp=1
  Data Type Conversion : DataTypeConversion  OutDataTypeStr=double
  MATLAB game1 : MATLAB Function  TreatAsAtomicUnit=on  SystemSampleTime=1
  MATLAB game2 : MATLAB Function  TreatAsAtomicUnit=on  SystemSampleTime=5
  Manual Switch : ManualSwitch
  Repeating Sequence : simulink/Sources/Repeating Sequence  rep_seq_t=[0 5]  rep_seq_y=[0 0.1]
  Saturation : Saturate  UpperLimit=50  LowerLimit=-50
  Saturation1 : Saturate  UpperLimit=0.9  LowerLimit=0.1
  Scope{2..7,9} (7 alike) : Scope
  Scope8 : Scope  NumInputPorts=2
  Switch : Switch  Criteria=u2 > Threshold  Threshold=0.05
  Switch1 : Switch  Criteria=u2 > Threshold  Threshold=-0.05
  Switch2 : Switch
  Unit Delay : UnitDelay
  Unit Delay1 : UnitDelay  SampleTime=0.1
  Unit Delay2 : UnitDelay  InitialCondition=0.5  SampleTime=5
  Zero-Order Hold : ZeroOrderHold
  Out1 : Outport
  Out2 : Outport  Port=2
  wires:
  MATLAB game2/2(alphao) -> Out2/1
  Data Type Conversion/1 -> MATLAB game2/6(t_int)
  MATLAB game2/1(k) -> Manual Switch/2, Scope9/1, Switch1/1, Add1/2, Switch/3, Add/2, Scope8/1
  In3/1 -> MATLAB game2/3(b0)
  In2/1 -> MATLAB game2/2(ti)
  In1/1 -> MATLAB game2/1(SoC)
  In5/1 -> MATLAB game2/4(phi)
  In4/1 -> MATLAB game2/5(label)
  In6/1 -> MATLAB game2/7(Energy)
  Counter Limited/1 -> Data Type Conversion/1
  Saturation/1 -> Unit Delay/1
  MATLAB game1/1(deadload) -> Saturation/1, Scope3/1
  In7/1 -> Unit Delay1/1
  Unit Delay1/1 -> Scope2/1, Zero-Order Hold/1, MATLAB game2/9(E)
  Repeating Sequence/1 -> MATLAB game1/3(decaytime)
  decay/1 -> MATLAB game1/4(decayfactor)
  Unit Delay2/1 -> Bias1/1, Add1/1, Add/1, Bias/1, Scope8/2
  Add/1 -> Scope6/1, Switch2/2, Switch/2
  Add1/1 -> Switch1/2
  Switch/1 -> Switch2/1, Scope5/1
  Switch1/1 -> Scope7/1, Switch2/3
  Switch2/1 -> Manual Switch/1, Unit Delay2/1, Saturation1/1
  Bias/1 -> Switch/1
  Bias1/1 -> Switch1/3
  Saturation1/1 -> Scope4/1
  Manual Switch/1 -> Out1/1
  Unit Delay/1 -> MATLAB game1/2(deadloadold)
  Zero-Order Hold/1 -> MATLAB game1/1(E)

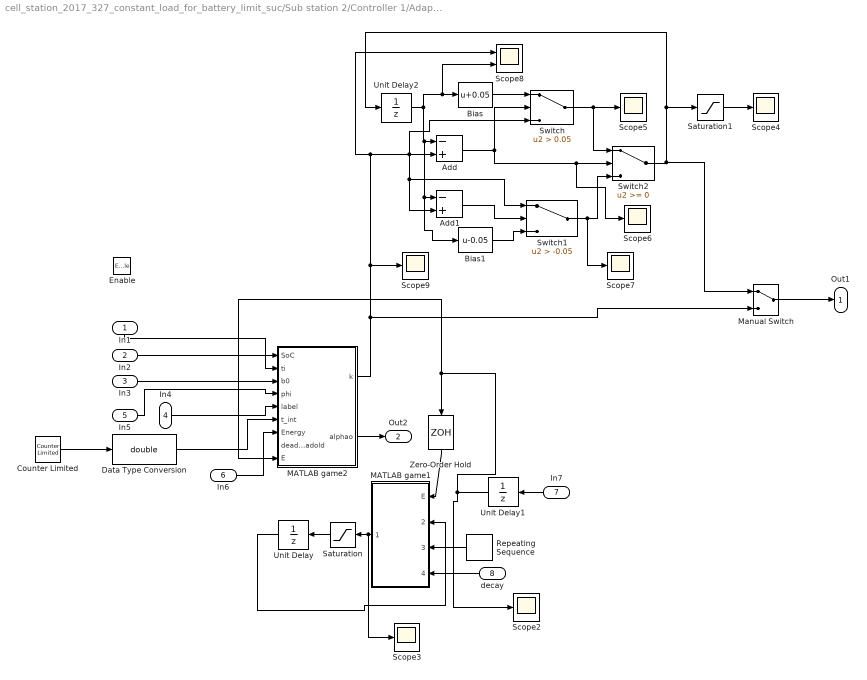
== system cell_station_2017_327_constant_load_for_battery_limit_suc/Sub station 2/Controller 1/Adaptive game solver/game solver ==
  In1 : Inport
  In2 : Inport  Port=2
  In3 : Inport  Port=3
  In4 : Inport  Port=4
  In5 : Inport  Port=5
  In6 : Inport  Port=6
  In7 : Inport  Port=7
  decay : Inport  Port=8
  Enable : EnablePort
  Add : Sum  Inputs=-+
  Add1 : Sum  Inputs=-+
  Bias : Bias  Bias=0.05
  Bias1 : Bias  Bias=-0.05
  Counter Limited : simulink/Sources/Counter Limited  uplimit=24  tsamp=1
  Data Type Conversion : DataTypeConversion  OutDataTypeStr=double
  MATLAB game1 : MATLAB Function  TreatAsAtomicUnit=on  SystemSampleTime=1
  MATLAB game2 : MATLAB Function  TreatAsAtomicUnit=on  SystemSampleTime=5
  Manual Switch : ManualSwitch
  Repeating Sequence : simulink/Sources/Repeating Sequence  rep_seq_t=[0 5]  rep_seq_y=[0 0.1]
  Saturation : Saturate  UpperLimit=50  LowerLimit=-50
  Saturation1 : Saturate  UpperLimit=0.9  LowerLimit=0.1
  Scope{2..7,9} (7 alike) : Scope
  Scope8 : Scope  NumInputPorts=2
  Switch : Switch  Criteria=u2 > Threshold  Threshold=0.05
  Switch1 : Switch  Criteria=u2 > Threshold  Threshold=-0.05
  Switch2 : Switch
  Unit Delay : UnitDelay
  Unit Delay1 : UnitDelay  SampleTime=0.1
  Unit Delay2 : UnitDelay  InitialCondition=0.5  SampleTime=5
  Zero-Order Hold : ZeroOrderHold
  Out1 : Outport
  Out2 : Outport  Port=2
  wires:
  MATLAB game2/2(alphao) -> Out2/1
  Data Type Conversion/1 -> MATLAB game2/6(t_int)
  MATLAB game2/1(k) -> Manual Switch/2, Scope9/1, Switch1/1, Add1/2, Switch/3, Add/2, Scope8/1
  In3/1 -> MATLAB game2/3(b0)
  In2/1 -> MATLAB game2/2(ti)
  In1/1 -> MATLAB game2/1(SoC)
  In5/1 -> MATLAB game2/4(phi)
  In4/1 -> MATLAB game2/5(label)
  In6/1 -> MATLAB game2/7(Energy)
  Counter Limited/1 -> Data Type Conversion/1
  Saturation/1 -> Unit Delay/1
  MATLAB game1/1(deadload) -> Saturation/1, Scope3/1
  In7/1 -> Unit Delay1/1
  Unit Delay1/1 -> Scope2/1, Zero-Order Hold/1, MATLAB game2/9(E)
  Repeating Sequence/1 -> MATLAB game1/3(decaytime)
  decay/1 -> MATLAB game1/4(decayfactor)
  Unit Delay2/1 -> Bias1/1, Add1/1, Add/1, Bias/1, Scope8/2
  Add/1 -> Scope6/1, Switch2/2, Switch/2
  Add1/1 -> Switch1/2
  Switch/1 -> Switch2/1, Scope5/1
  Switch1/1 -> Scope7/1, Switch2/3
  Switch2/1 -> Manual Switch/1, Unit Delay2/1, Saturation1/1
  Bias/1 -> Switch/1
  Bias1/1 -> Switch1/3
  Saturation1/1 -> Scope4/1
  Manual Switch/1 -> Out1/1
  Unit Delay/1 -> MATLAB game1/2(deadloadold)
  Zero-Order Hold/1 -> MATLAB game1/1(E)

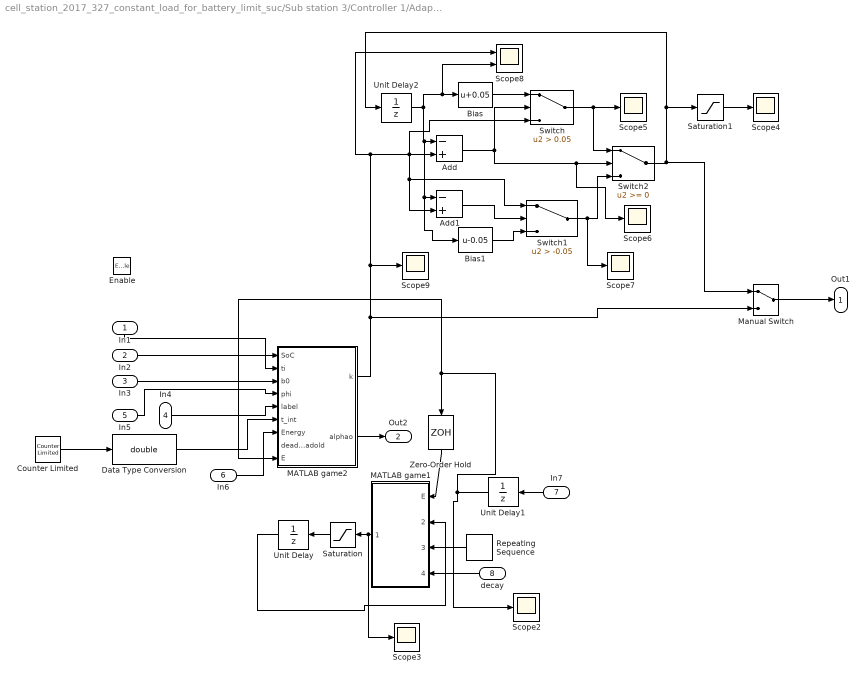
== system cell_station_2017_327_constant_load_for_battery_limit_suc/Sub station 3/Controller 1/Adaptive game solver/game solver ==
  In1 : Inport
  In2 : Inport  Port=2
  In3 : Inport  Port=3
  In4 : Inport  Port=4
  In5 : Inport  Port=5
  In6 : Inport  Port=6
  In7 : Inport  Port=7
  decay : Inport  Port=8
  Enable : EnablePort
  Add : Sum  Inputs=-+
  Add1 : Sum  Inputs=-+
  Bias : Bias  Bias=0.05
  Bias1 : Bias  Bias=-0.05
  Counter Limited : simulink/Sources/Counter Limited  uplimit=24  tsamp=1
  Data Type Conversion : DataTypeConversion  OutDataTypeStr=double
  MATLAB game1 : MATLAB Function  TreatAsAtomicUnit=on  SystemSampleTime=1
  MATLAB game2 : MATLAB Function  TreatAsAtomicUnit=on  SystemSampleTime=5
  Manual Switch : ManualSwitch
  Repeating Sequence : simulink/Sources/Repeating Sequence  rep_seq_t=[0 5]  rep_seq_y=[0 0.1]
  Saturation : Saturate  UpperLimit=50  LowerLimit=-50
  Saturation1 : Saturate  UpperLimit=0.9  LowerLimit=0.1
  Scope{2..7,9} (7 alike) : Scope
  Scope8 : Scope  NumInputPorts=2
  Switch : Switch  Criteria=u2 > Threshold  Threshold=0.05
  Switch1 : Switch  Criteria=u2 > Threshold  Threshold=-0.05
  Switch2 : Switch
  Unit Delay : UnitDelay
  Unit Delay1 : UnitDelay  SampleTime=0.1
  Unit Delay2 : UnitDelay  InitialCondition=0.5  SampleTime=5
  Zero-Order Hold : ZeroOrderHold
  Out1 : Outport
  Out2 : Outport  Port=2
  wires:
  MATLAB game2/2(alphao) -> Out2/1
  Data Type Conversion/1 -> MATLAB game2/6(t_int)
  MATLAB game2/1(k) -> Manual Switch/2, Scope9/1, Switch1/1, Add1/2, Switch/3, Add/2, Scope8/1
  In3/1 -> MATLAB game2/3(b0)
  In2/1 -> MATLAB game2/2(ti)
  In1/1 -> MATLAB game2/1(SoC)
  In5/1 -> MATLAB game2/4(phi)
  In4/1 -> MATLAB game2/5(label)
  In6/1 -> MATLAB game2/7(Energy)
  Counter Limited/1 -> Data Type Conversion/1
  Saturation/1 -> Unit Delay/1
  MATLAB game1/1(deadload) -> Saturation/1, Scope3/1
  In7/1 -> Unit Delay1/1
  Unit Delay1/1 -> Scope2/1, Zero-Order Hold/1, MATLAB game2/9(E)
  Repeating Sequence/1 -> MATLAB game1/3(decaytime)
  decay/1 -> MATLAB game1/4(decayfactor)
  Unit Delay2/1 -> Bias1/1, Add1/1, Add/1, Bias/1, Scope8/2
  Add/1 -> Scope6/1, Switch2/2, Switch/2
  Add1/1 -> Switch1/2
  Switch/1 -> Switch2/1, Scope5/1
  Switch1/1 -> Scope7/1, Switch2/3
  Switch2/1 -> Manual Switch/1, Unit Delay2/1, Saturation1/1
  Bias/1 -> Switch/1
  Bias1/1 -> Switch1/3
  Saturation1/1 -> Scope4/1
  Manual Switch/1 -> Out1/1
  Unit Delay/1 -> MATLAB game1/2(deadloadold)
  Zero-Order Hold/1 -> MATLAB game1/1(E)

== matlab function cell_station_2017_327_constant_load_for_battery_limit_suc/Sub station 1/Controller 1/Adaptive game solver/MATLAB game1 ==
  data: ti input; sitaguess output; phi input; label input; SoC input; SoC_old input; E output; alphao input; kself input; Estar output; sampletime input; E_aux input; Energy input
function [sitaguess,E,Estar] = multipleload(ti,phi,label,SoC,SoC_old,alphao,kself,sampletime,E_aux,Energy)
if SoC_old>0.1
p0=10;
t=ti/5;
rate=[0.1 0.4 0.5];

E=load2nojump(t)*rate(label)*kself+load2nojump(t)*(1-rate(label))*alphao(label)-solarnojump(t)*(solarnojump(t)>0)+p0*phi;
% sampletime=0.2;
% Estar=-(SoC-SoC_old)*Energy/sampletime;
Estar=-E_aux*Energy;
if abs(Estar)>48*360
    Estar=0;
end
 e0=E-Estar;
% e0=E-po;
sitaguess=0.5e-1*(e0*p0);
else
sitaguess=0;
E=0;
Estar=0;
e0=0;
end
end
%  
% function Pload=load2nojump(t)
% pl1 =    0.000839 ;
% pl2 =       1.205  ;
% pl3 =      -12.02 ;
% pl4 =       34.29  ;
% ql1 =      -6.495  ;
% ql2 =       43.45  ;
% Pload =max(0,(30* (pl1*(t).^3 + pl2*(t).^2 + pl3*(t) + pl4) ./((t).^2 + ql1*(t) + ql2))*(1+(0.2*rand-0.2*rand)*0));
% end


% 
% function [ko,koreal,alphao, kself] = gamesolver_virtual_load2(t_int,v,t,~,b0,batterystage,Energy,amin,daygoal,phi,sitenumber,rate,operation)
% alphao=zeros(1,sitenumber);
% kself=zeros(1,sitenumber);
% SoC=(v-56)*0.05+0.5;
% daygoal2=daygoal*batterystage;
% T=1;
% n=20;
% dT=T/n;
% realp=zeros(1,9);
% coder.extrinsic('linearprograming')
% coder.varsize('cost1','cost2','realrow','realcolumn')
% decide=zeros(1,sitenumber);
% P=zeros(1,batterystage*1.5);
% p=zeros(1,9);
% po=zeros(1,9);
% for ppt=1:sitenumber
%     if operation(ppt)~=0
%     opteva=zeros(9);
%     cost1=zeros(9);  
%     loadrate=rate(ppt);
% for k0=amin:1:9
%  for sigmaother0=amin:1:9
%         k=k0*0.1;
%         sigmaother=sigmaother0*0.1;       
%         [En,Sn]=pdf2_virtual_load(t,dT,loadrate,k,sigmaother,n*(24-t_int),phi(ppt));
%         if t_int~=24
%         for l=1:(batterystage*1.5)
%         P(l)=normcdf(((Energy/batterystage*(l+1)-SoC*Energy)-En*(24-t_int))/sqrt(Sn))-(normcdf(((Energy/batterystage*(l)-SoC*Energy)-En*(24-t_int))/sqrt(Sn)));
%         end
%         if (1-sum(P(1:daygoal2)))>0.5 %if there is  possibility reaching 0.8 SoC?
%             opteva(k0,sigmaother0)=b0*(sum(P(daygoal2:end)));
%             cost1(k0,sigmaother0)=((k*loadrate+sigmaother*(1-loadrate))*(1-b0)*SoC+opteva(k0,sigmaother0));
%         else  %if not stay at minimum alpha
%             cost1(k0,sigmaother0)=(1-k)/10;
%         end
%         else
%             cost1(k0,sigmaother0)=(k*loadrate+sigmaother*(1-loadrate))*(1-b0)+b0*SoC;
%         end
%  end
% end
%  [m,~]=size(cost1);
%  realrow=1:m;
% p(1:amin-1)=0;
% p(amin:9)=linearprograming(cost1(amin:9,amin:9))';
% po(1:amin-1)=0;
% po(amin:9)=linearprograming(cost1(amin:9,amin:9)')';
% linespace=0.1:0.1:0.9;
% alphao(ppt)=po*linespace';
% realn=size(realrow,2);
% for i=1:realn    
%     realp(realrow(i))=p(i);
% end
% r=rand;
% l=0;
% for i=1:9        
%     l=l+realp(i);
%     if l>r
%         break
%     end
% end
% decide(ppt)=i*0.1; 
%     end
% end
% kself=decide;
% ko=decide*rate(1:sitenumber)'/sum(rate(1:sitenumber));
% koreal=decide*rate(1:sitenumber)';
% end

== matlab function cell_station_2017_327_constant_load_for_battery_limit_suc/Environment/MATLAB Function2 ==
  data: x input; y output
function y = fcn(x)
%#codegen
p1 =      -327.4 ;
p2 =   4.435e+04;
p3 =  -7.078e+05;
q1 =      -143.6 ;
q2 =        5928 ;
f = (p1*x^2 + p2*x + p3) / (x^2 + q1*x + q2)/2;
y = f;

== matlab function cell_station_2017_327_constant_load_for_battery_limit_suc/Environment/MATLAB Function1 ==
  data: x input; y output
function y = fcn(x)
%#codegen

       p1 =    0.000839 ;
       p2 =       1.205  ;
       p3 =      -12.02 ;
       p4 =       34.29  ;
       q1 =      -6.495 ;
       q2 =       43.45 ;
       f = (p1*x^3 + p2*x^2 + p3*x + p4) /(x^2 + q1*x + q2);

y = f;

== matlab function cell_station_2017_327_constant_load_for_battery_limit_suc/Sub station 1/Controller 1/Adaptive game solver/game solver/MATLAB game1 ==
  data: E input; deadload output; deadloadold input; decaytime input; decayfactor input
function deadload  = decay(E,deadloadold,decaytime,decayfactor)
deadload=deadloadold;
power=E;
if power>100
    deadload=power;
elseif power<-100
    deadload=power;
elseif power+deadload>100||power+deadload<-100
    deadload=deadloadold;
else
    deadload=deadloadold*exp(decayfactor*decaytime);
end
end

== matlab function cell_station_2017_327_constant_load_for_battery_limit_suc/Sub station 2/Controller 1/Adaptive game solver/MATLAB game1 ==
  data: ti input; sitaguess output; phi input; label input; SoC input; SoC_old input; E output; alphao input; kself input; Estar output; sampletime input; E_aux input; Energy input
function [sitaguess,E,Estar] = multipleload(ti,phi,label,SoC,SoC_old,alphao,kself,sampletime,E_aux,Energy)
if SoC_old>0.1
p0=10;
t=ti/5;
rate=[0.1 0.4 0.5];

E=load2nojump(t)*rate(label)*kself+load2nojump(t)*(1-rate(label))*alphao(label)-solarnojump(t)*(solarnojump(t)>0)+p0*phi;
% sampletime=0.2;
% Estar=-(SoC-SoC_old)*Energy/sampletime;
Estar=-E_aux*Energy;
if abs(Estar)>48*360
    Estar=0;
end
 e0=E-Estar;
% e0=E-po;
sitaguess=0.5e-1*(e0*p0);
else
sitaguess=0;
E=0;
Estar=0;
e0=0;
end
end
%  
% function Pload=load2nojump(t)
% pl1 =    0.000839 ;
% pl2 =       1.205  ;
% pl3 =      -12.02 ;
% pl4 =       34.29  ;
% ql1 =      -6.495  ;
% ql2 =       43.45  ;
% Pload =max(0,(30* (pl1*(t).^3 + pl2*(t).^2 + pl3*(t) + pl4) ./((t).^2 + ql1*(t) + ql2))*(1+(0.2*rand-0.2*rand)*0));
% end


% 
% function [ko,koreal,alphao, kself] = gamesolver_virtual_load2(t_int,v,t,~,b0,batterystage,Energy,amin,daygoal,phi,sitenumber,rate,operation)
% alphao=zeros(1,sitenumber);
% kself=zeros(1,sitenumber);
% SoC=(v-56)*0.05+0.5;
% daygoal2=daygoal*batterystage;
% T=1;
% n=20;
% dT=T/n;
% realp=zeros(1,9);
% coder.extrinsic('linearprograming')
% coder.varsize('cost1','cost2','realrow','realcolumn')
% decide=zeros(1,sitenumber);
% P=zeros(1,batterystage*1.5);
% p=zeros(1,9);
% po=zeros(1,9);
% for ppt=1:sitenumber
%     if operation(ppt)~=0
%     opteva=zeros(9);
%     cost1=zeros(9);  
%     loadrate=rate(ppt);
% for k0=amin:1:9
%  for sigmaother0=amin:1:9
%         k=k0*0.1;
%         sigmaother=sigmaother0*0.1;       
%         [En,Sn]=pdf2_virtual_load(t,dT,loadrate,k,sigmaother,n*(24-t_int),phi(ppt));
%         if t_int~=24
%         for l=1:(batterystage*1.5)
%         P(l)=normcdf(((Energy/batterystage*(l+1)-SoC*Energy)-En*(24-t_int))/sqrt(Sn))-(normcdf(((Energy/batterystage*(l)-SoC*Energy)-En*(24-t_int))/sqrt(Sn)));
%         end
%         if (1-sum(P(1:daygoal2)))>0.5 %if there is  possibility reaching 0.8 SoC?
%             opteva(k0,sigmaother0)=b0*(sum(P(daygoal2:end)));
%             cost1(k0,sigmaother0)=((k*loadrate+sigmaother*(1-loadrate))*(1-b0)*SoC+opteva(k0,sigmaother0));
%         else  %if not stay at minimum alpha
%             cost1(k0,sigmaother0)=(1-k)/10;
%         end
%         else
%             cost1(k0,sigmaother0)=(k*loadrate+sigmaother*(1-loadrate))*(1-b0)+b0*SoC;
%         end
%  end
% end
%  [m,~]=size(cost1);
%  realrow=1:m;
% p(1:amin-1)=0;
% p(amin:9)=linearprograming(cost1(amin:9,amin:9))';
% po(1:amin-1)=0;
% po(amin:9)=linearprograming(cost1(amin:9,amin:9)')';
% linespace=0.1:0.1:0.9;
% alphao(ppt)=po*linespace';
% realn=size(realrow,2);
% for i=1:realn    
%     realp(realrow(i))=p(i);
% end
% r=rand;
% l=0;
% for i=1:9        
%     l=l+realp(i);
%     if l>r
%         break
%     end
% end
% decide(ppt)=i*0.1; 
%     end
% end
% kself=decide;
% ko=decide*rate(1:sitenumber)'/sum(rate(1:sitenumber));
% koreal=decide*rate(1:sitenumber)';
% end
